simulink model "parity_generator_checker_3bit"  (R2025b)
settings: Solver=VariableStepAuto  StartTime=0.0  StopTime=10.0  RelTol=1e-3
settings Model: Creator=Johan  LastModifiedBy=Johan

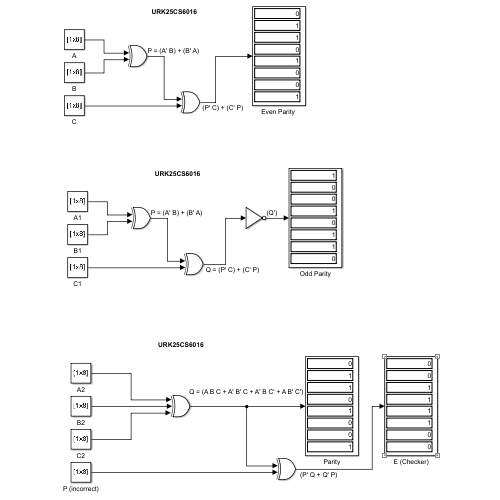
[thumbnail: Simulink's stored preview of the top-level diagram]
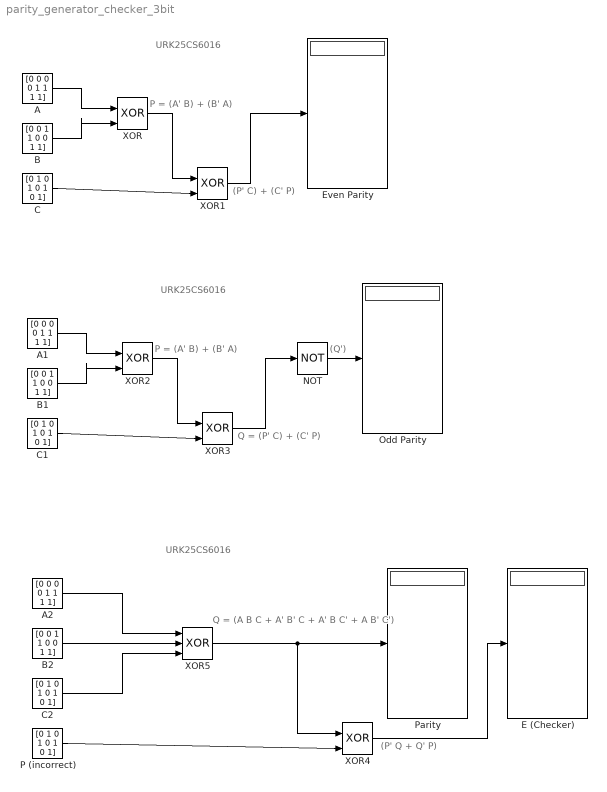
== system parity_generator_checker_3bit ==
  note: (P' Q + Q' P)
  note: (Q')
  note: P = (A' B) + (B' A)
  note: (P' C) + (C' P)
  note: URK25CS6016
  note: P = (A' B) + (B' A)
  note: Q = (P' C) + (C' P)
  note: URK25CS6016
  note: Q = (A B C + A' B' C + A' B C' + A B' C')
  note: URK25CS6016
  A : Constant  Value=[0 0 0 0 1 1 1 1]
  A1 : Constant  Value=[0 0 0 0 1 1 1 1]
  A2 : Constant  Value=[0 0 0 0 1 1 1 1]
  B : Constant  Value=[0 0 1 1 0 0 1 1]
  B1 : Constant  Value=[0 0 1 1 0 0 1 1]
  B2 : Constant  Value=[0 0 1 1 0 0 1 1]
  C : Constant  Value=[0 1 0 1 0 1 0 1]
  C1 : Constant  Value=[0 1 0 1 0 1 0 1]
  C2 : Constant  Value=[0 1 0 1 0 1 0 1]
  E (Checker) : Display
  "Even Parity " : Display
  NOT : Logic  Operator=NOT  IconShape=distinctive  AllPortsSameDT=off  OutDataTypeStr=boolean
  Odd Parity : Display
  P (incorrect) : Constant  Value=[0 1 0 1 0 1 0 1]
  Parity : Display
  XOR{,1..4} (5 alike) : Logic  Operator=XOR  IconShape=distinctive  AllPortsSameDT=off  OutDataTypeStr=boolean
  XOR5 : Logic  Operator=XOR  Inputs=3  IconShape=distinctive  AllPortsSameDT=off  OutDataTypeStr=boolean
  wires:
  A/1 -> XOR/1
  B/1 -> XOR/2
  C/1 -> XOR1/2
  XOR/1 -> XOR1/1
  XOR1/1 -> "Even Parity "/1
  XOR2/1 -> XOR3/1
  C1/1 -> XOR3/2
  B1/1 -> XOR2/2
  A1/1 -> XOR2/1
  NOT/1 -> Odd Parity/1
  XOR3/1 -> NOT/1
  A2/1 -> XOR5/1
  B2/1 -> XOR5/2
  C2/1 -> XOR5/3
  XOR5/1 -> XOR4/1, Parity/1
  XOR4/1 -> E (Checker)/1
  P (incorrect)/1 -> XOR4/2
